simulink model "lab_9_unkown_decoupling"  (R2023a)
settings: Solver=VariableStepAuto  StartTime=0.0  StopTime=10  RelTol=1e-3
values from neighbouring files (symbols this model uses):
  A = eye(3) + Ts * A    [part_deriv.m]
undefined symbols (not defined in the file or in its folder): B, C, Ce, E, Ke, x10, x20, x30
settings Model: Creator=bz  LastModifiedBy=bz

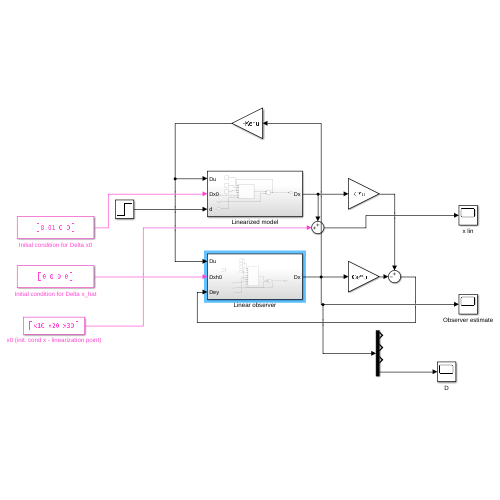
[thumbnail: Simulink's stored preview of the top-level diagram]
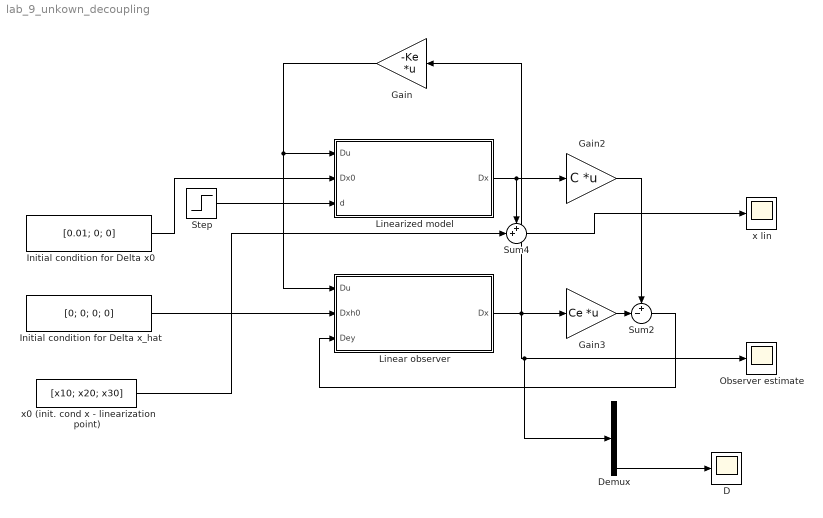
== system lab_9_unkown_decoupling ==
  D : Scope
  Demux : Demux
  Gain : Gain  Gain=-Ke  Multiplication=Matrix(K*u)
  Gain2 : Gain  Gain=C  Multiplication=Matrix(K*u)
  Gain3 : Gain  Gain=Ce  Multiplication=Matrix(K*u)
  Initial condition for Delta x0 : Constant  Value=[0.01; 0; 0]
  Initial condition for Delta x_hat : Constant  Value=[0; 0; 0; 0]
  Linear observer : Subsystem
  Linearized model : Subsystem
  Observer estimate : Scope
  Step : Step  Time=3  SampleTime=0
  Sum2 : Sum  Inputs=+-|
  Sum4 : Sum  Inputs=++|
  x lin : Scope
  x0 (init. cond x - linearization point) : Constant  Value=[x10; x20; x30]
  wires:
  Initial condition for Delta x0/1 -> Linearized model/2(Dx0)
  x0 (init. cond x - linearization point)/1 -> Sum4/2
  Gain/1 -> Linear observer/1(Du), Linearized model/1(Du)
  Linearized model/1(Dx) -> Gain2/1, Sum4/1
  Linear observer/1(Dx) -> Demux/1, Observer estimate/1, Gain3/1, Gain/1
  Initial condition for Delta x_hat/1 -> Linear observer/2(Dxh0)
  Sum2/1 -> Linear observer/3(Dey)
  Gain2/1 -> Sum2/1
  Gain3/1 -> Sum2/2
  Sum4/1 -> x lin/1
  Demux/4 -> D/1
  Step/1 -> Linearized model/3(d)

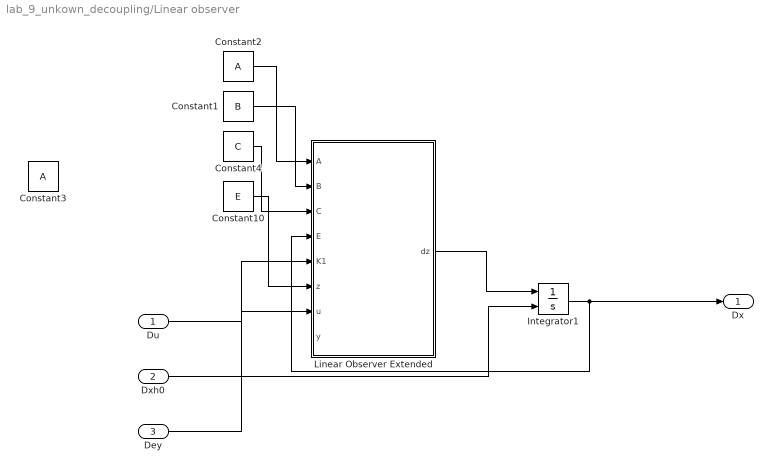
== system lab_9_unkown_decoupling/Linear observer ==
  Du : Inport
  Dxh0 : Inport  Port=2
  Dey : Inport  Port=3
  Constant1 : Constant  Value=B
  Constant10 : Constant  Value=E
  Constant2 : Constant  Value=A
  Constant3 : Constant  Value=A
  Constant4 : Constant  Value=C
  Integrator1 : Integrator  InitialConditionSource=external
  Linear Observer Extended : MATLAB Function  TreatAsAtomicUnit=on
  Dx : Outport
  wires:
  Linear Observer Extended/1(dz) -> Integrator1/1
  Integrator1/1 -> Dx/1, Linear Observer Extended/4(E)
  Dxh0/1 -> Integrator1/2
  Du/1 -> Linear Observer Extended/7(u)
  Dey/1 -> Linear Observer Extended/5(K1)
  Constant4/1 -> Linear Observer Extended/3(C)
  Constant1/1 -> Linear Observer Extended/2(B)
  Constant2/1 -> Linear Observer Extended/1(A)
  Constant10/1 -> Linear Observer Extended/6(z)

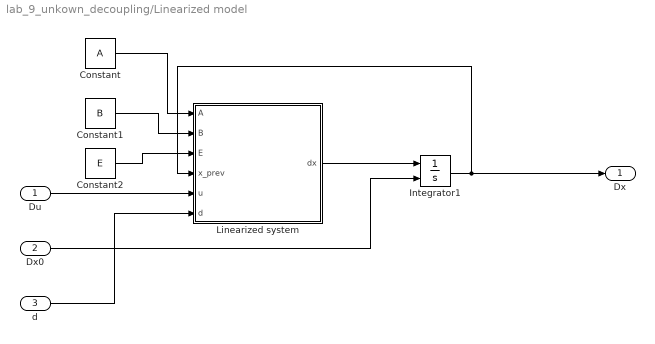
== system lab_9_unkown_decoupling/Linearized model ==
  Du : Inport
  Dx0 : Inport  Port=2
  d : Inport  Port=3
  Constant : Constant  Value=A
  Constant1 : Constant  Value=B
  Constant2 : Constant  Value=E
  Integrator1 : Integrator  InitialConditionSource=external
  Linearized system : MATLAB Function  TreatAsAtomicUnit=on
  Dx : Outport
  wires:
  Linearized system/1(dx) -> Integrator1/1
  Integrator1/1 -> Dx/1, Linearized system/4(x_prev)
  Dx0/1 -> Integrator1/2
  Du/1 -> Linearized system/5(u)
  Constant/1 -> Linearized system/1(A)
  Constant1/1 -> Linearized system/2(B)
  Constant2/1 -> Linearized system/3(E)
  d/1 -> Linearized system/6(d)

== matlab function lab_9_unkown_decoupling/Linearized model/Linearized system ==
  data: A input; B input; E input; x_prev input; u input; dx output size=[3,1]; d input
function dx = fcn(A, B, E, x_prev, u, d)

dx = A * x_prev + B * u + E * d;

end

== matlab function lab_9_unkown_decoupling/Linear observer/Linear Observer Extended ==
  data: A input; B input; C input; E input; K1 input; z input; u input; dz output; y input
function dz = fcn(A, B, C, E, K1, z, u, y)

H = E * pinv(C*E);
T = eye(4) - H * C;

F = T*A - K1*C;
K2 = F*H;

K = K1 + K2;

dz = F*z + T*B*u + K*y;

end
